simulink library "rotorTorqueCtrlDiscrete"  (R2022a)
settings: Solver=VariableStepAuto  StartTime=0.0  StopTime=10.0  RelTol=1e-3
undefined symbols (not defined in the file): rho, vhcl
settings Model: Creator=adabney  LastModifiedBy=adabney

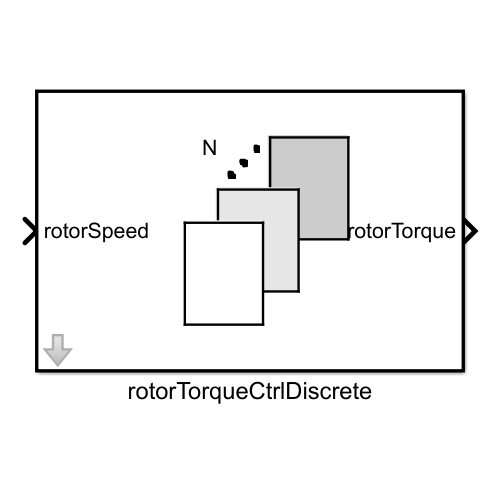
[thumbnail: Simulink's stored preview of the top-level diagram]
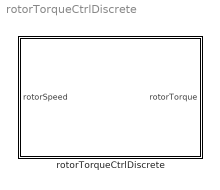
== system rotorTorqueCtrlDiscrete ==
  rotorTorqueCtrlDiscrete : Subsystem  TreatAsAtomicUnit=on  mask{turb_struct=vhcl.struct('OCT.turb'), rho=rho}
      mask prompts: turb_struct "Turbine Structures"; rho "Fluid Density"

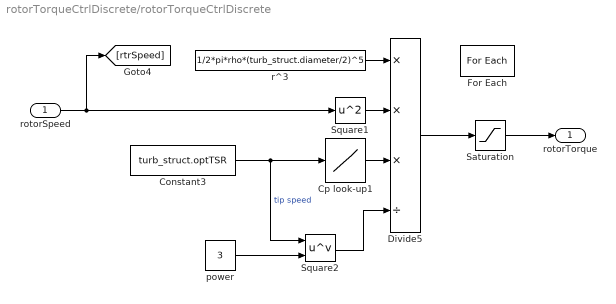
== system rotorTorqueCtrlDiscrete/rotorTorqueCtrlDiscrete ==
  rotorSpeed : Inport  Partition=on  PartitionDimension=1  PartitionWidth=1  PartitionOffset=0
  Constant3 : Constant  Value=turb_struct.optTSR
  Cp look-up1 : Lookup_n-D  NumberOfTableDimensions=1  BreakpointsForDimension1=turb_struct.RPMref  Table=turb_struct.CpLookup  InternalRulePriority=Speed  RndMeth=Simplest
  Divide5 : Product  Inputs=***/
  For Each : ForEach  DisableCoverage=on  IterateSubsysMaskParameter=on,off  SubsysMaskParameterIterationDimension=2,1  SubsysMaskParameterIterationStepSize=1,1
  Saturation : Saturate  UpperLimit=42  LowerLimit=-42
  Square1 : Math  Operator=square
  Square2 : Math  Operator=pow
  power : Constant  Value=3
  r^3 : Constant  Value=1/2*pi*rho*(turb_struct.diameter/2)^5
  rotorTorque : Outport  ConcatenationDimension=1
  wires:
  power/1 -> Square2/2
  Cp look-up1/1 -> Divide5/3
  Square1/1 -> Divide5/2
  Square2/1 -> Divide5/4
  r^3/1 -> Divide5/1
  Constant3/1 -> Square2/1, Cp look-up1/1  "tip speed"
  rotorSpeed/1 -> [rtrSpeed], Square1/1
  Saturation/1 -> rotorTorque/1
  Divide5/1 -> Saturation/1
